simulink model "Boat_sim_HeadingHold"  (Simulink 7.5)
settings: Solver=FixedStepDiscrete  StartTime=0.0  StopTime=1000  FixedStep=.01  RelTol=1e-3
InitFcn:
  | boat_constants
values from neighbouring files (symbols this model uses):
  C_d_sea_surge = 340    [boat_constants.m]
  d_prop = .4572    (= 0.4572)    [boat_constants.m]
  figure8_waypoints = int32([ ... (first row only)    [boat_constants.m]
  K_t = 0.5    [boat_constants.m]
  mass = 550    [boat_constants.m]
  OC2max = 49999    [boat_constants.m]    (also in simulation_constants.m)
  phi_0 = 0    [boat_constants.m]    (also in simulation_constants.m)
  rho_w = 1.03e3    (= 1030)    [boat_constants.m]
  sampling_waypoints = int32([ ... (first row only)    [boat_constants.m]
  T_step = 0.01    [boat_constants.m]    (also in common.m)
  test_waypoints = int32([ ... (first row only)    [boat_constants.m]
  wheelbase = 3.27    [boat_constants.m]
undefined symbols (not defined in the file or in its folder): clock, DiscIntNeverNeededParam, Earth, WGS84
libraries: simulink x24, uSimLib x6, instrumentlib x2, aerolibconvert2 x2, aerolibtransform2 x1, aerolibanimutils x1, simulink_need_slupdate x1
(part 1 of 2)
settings Model: Creator=Administrator  LastModifiedBy=Bryant  ExtModeAutoUpdateStatusClock=off  BufferReuse=off
settings DataIOCC: MaxDataPoints=1  SaveOutput=off  SignalLogging=off  DSMLogging=off
settings OptimizationCC: BlockReduction=off  InlineParams=on  UseIntDivNetSlope=on  InlineInvariantSignals=on  BufferReuse=off  InitFltsAndDblsToZero=on  EfficientFloat2IntCast=on  SimCompilerOptimization=On
settings DebuggingCC: ReadBeforeWriteMsg=DisableAll  SaveWithParameterizedLinksMsg=none  FcnCallInpInsideContextMsg=Enable All  UniqueDataStoreMsg=error  AssertControl=DisableAll  StrictBusMsg=Warning
settings HardwareCC: ProdBitPerInt=16  ProdIntDivRoundTo=Zero  ProdEndianess=LittleEndian  ProdWordSize=16  ProdHWDeviceType=Microchip->dsPIC
settings GRTTargetCC: TargetFcnLib=ansi_tfl_tmw.mat

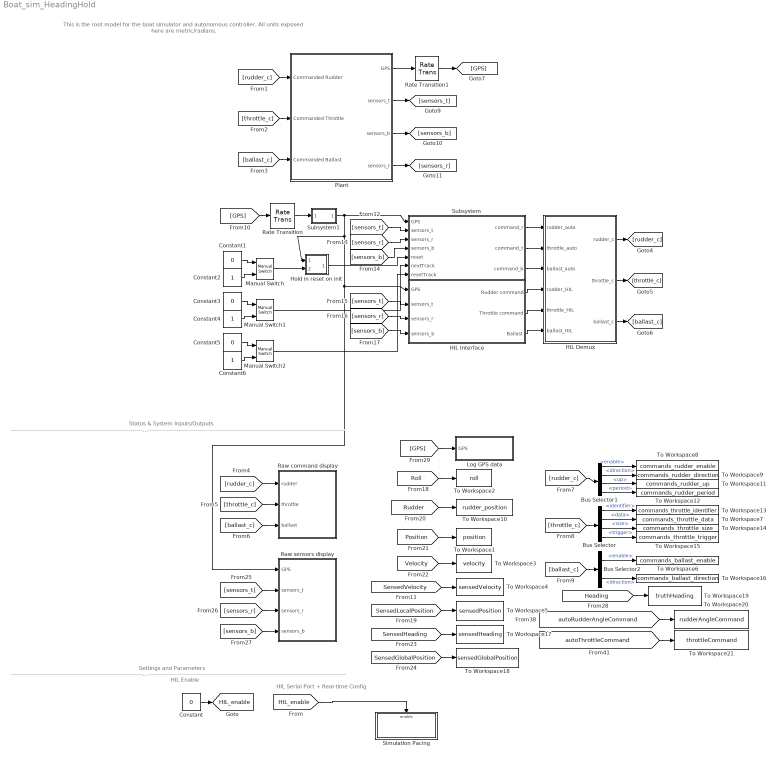
== system Boat_sim_HeadingHold ==
  note: This is the root model for the boat simulator and autonomous controller. All
      | units exposed here are metric/radians.
  note: HIL Enable
  note: Settings and Parameters
      | ---------------------------------------------------------------------------------------------------------------------------------------------------------------------------------------------------------------------------------------------------------
  note: HIL Serial Port + Real-time Config
  note: Status & System Inputs/Outputs
      | ---------------------------------------------------------------------------------------------------------------------------------------------------------------------------------------------------------------------------------------------------------
  Bus Selector : BusSelector  OutputSignals=identifier,data,size,trigger
  Bus Selector1 : BusSelector  OutputSignals=enable,direction,up,period
  Bus Selector2 : BusSelector  OutputSignals=enable,direction
  Constant : Constant  Value=0  OutDataTypeMode=boolean  OutDataType=fixdt(1, 16)  OutScaling=2^0  OutDataTypeStr=boolean
  Constant1 : Constant  Value=0  OutDataTypeMode=boolean  OutDataType=fixdt(1, 16)  OutScaling=2^0  OutDataTypeStr=boolean  SampleTime=Inf
  Constant2 : Constant  OutDataTypeMode=boolean  OutDataType=fixdt(1, 16)  OutScaling=2^0  OutDataTypeStr=boolean  SampleTime=Inf
  Constant3 : Constant  Value=0  OutDataTypeMode=boolean  OutDataType=fixdt(1, 16)  OutScaling=2^0  OutDataTypeStr=boolean  SampleTime=Inf
  Constant4 : Constant  OutDataTypeMode=boolean  OutDataType=fixdt(1, 16)  OutScaling=2^0  OutDataTypeStr=boolean  SampleTime=Inf
  Constant5 : Constant  Value=0  OutDataTypeMode=boolean  OutDataType=fixdt(1, 16)  OutScaling=2^0  OutDataTypeStr=boolean  SampleTime=Inf
  Constant6 : Constant  OutDataTypeMode=boolean  OutDataType=fixdt(1, 16)  OutScaling=2^0  OutDataTypeStr=boolean  SampleTime=Inf
  HIL Demux : Subsystem
  HIL Interface : Subsystem
  Hold in reset on init : Subsystem
  Log GPS data : Subsystem
  Manual Switch : simulink/Signal Routing/Manual Switch  SystemSampleTime=-1  sw=1  action=0  varsize=off
  Manual Switch1 : simulink/Signal Routing/Manual Switch  SystemSampleTime=-1  sw=1  action=0  varsize=off
  Manual Switch2 : simulink/Signal Routing/Manual Switch  SystemSampleTime=-1  sw=1  action=0  varsize=off
  Plant : Subsystem
  Rate Transition : RateTransition  Deterministic=off
  Rate Transition1 : RateTransition  Deterministic=off  OutPortSampleTime=1
  Raw command display : Subsystem
  Raw sensors display : Subsystem
  Simulation Pacing : Subsystem  TreatAsAtomicUnit=on
  Subsystem : Subsystem
  Subsystem1 : Subsystem
  To Workspace1 : ToWorkspace  VariableName=position  SampleTime=-1  SaveFormat=Array
  To Workspace10 : ToWorkspace  VariableName=rudder_position  SampleTime=-1  SaveFormat=Array
  To Workspace11 : ToWorkspace  VariableName=commands_rudder_up  SampleTime=-1  SaveFormat=Array
  To Workspace12 : ToWorkspace  VariableName=commands_rudder_period  SampleTime=-1  SaveFormat=Array
  To Workspace13 : ToWorkspace  VariableName=commands_throttle_identifier  SampleTime=-1  SaveFormat=Array
  To Workspace14 : ToWorkspace  VariableName=commands_throttle_size  SampleTime=-1  SaveFormat=Array
  To Workspace15 : ToWorkspace  VariableName=commands_throttle_trigger  SampleTime=-1  SaveFormat=Array
  To Workspace16 : ToWorkspace  VariableName=commands_ballast_direction  SampleTime=-1  SaveFormat=Array
  To Workspace17 : ToWorkspace  VariableName=sensedHeading  SampleTime=-1  SaveFormat=Array
  To Workspace18 : ToWorkspace  VariableName=sensedGlobalPosition  SampleTime=-1  SaveFormat=Array
  To Workspace19 : ToWorkspace  VariableName=truthHeading  SampleTime=-1  SaveFormat=Array
  To Workspace2 : ToWorkspace  VariableName=roll  SampleTime=-1  SaveFormat=Array
  To Workspace20 : ToWorkspace  VariableName=rudderAngleCommand  SampleTime=-1  SaveFormat=Array
  To Workspace21 : ToWorkspace  VariableName=throttleCommand  SampleTime=-1  SaveFormat=Array
  To Workspace3 : ToWorkspace  VariableName=velocity  SampleTime=-1  SaveFormat=Array
  To Workspace4 : ToWorkspace  VariableName=sensedVelocity  SampleTime=-1  SaveFormat=Array
  To Workspace5 : ToWorkspace  VariableName=sensedPosition  SampleTime=-1  SaveFormat=Array
  To Workspace6 : ToWorkspace  VariableName=commands_ballast_enable  SampleTime=-1  SaveFormat=Array
  To Workspace7 : ToWorkspace  VariableName=commands_throttle_data  SampleTime=-1  SaveFormat=Array
  To Workspace8 : ToWorkspace  VariableName=commands_rudder_enable  SampleTime=-1  SaveFormat=Array
  To Workspace9 : ToWorkspace  VariableName=commands_rudder_direction  SampleTime=-1  SaveFormat=Array
  tag scope: HIL_enable=global
  wires:
  Plant/4(sensors_r) -> [sensors_r]
  Constant/1 -> [HIL_enable]
  Subsystem/1(command_r) -> HIL Demux/1(rudder_auto)
  Subsystem/2(command_t) -> HIL Demux/2(throttle_auto)
  Subsystem/3(command_b) -> HIL Demux/3(ballast_auto)
  [rudder_c] -> Plant/1(Commanded Rudder)
  [throttle_c] -> Plant/2(Commanded Throttle)
  [ballast_c] -> Plant/3(Commanded Ballast)
  Plant/1(GPS) -> Rate Transition1/1
  Plant/3(sensors_b) -> [sensors_b]
  Plant/2(sensors_t) -> [sensors_t]
  [sensors_b] -> Subsystem/4(sensors_b)
  [sensors_r] -> Subsystem/3(sensors_r)
  [sensors_t] -> Subsystem/2(sensors_t)
  Constant1/1 -> Manual Switch/1
  Constant2/1 -> Manual Switch/2
  [rudder_c] -> Raw command display/1(rudder)
  [throttle_c] -> Raw command display/2(throttle)
  [ballast_c] -> Raw command display/3(ballast)
  [sensors_t] -> Raw sensors display/2(sensors_t)
  [sensors_r] -> Raw sensors display/3(sensors_r)
  [sensors_b] -> Raw sensors display/4(sensors_b)
  HIL Interface/1(Rudder command) -> HIL Demux/4(rudder_HIL)
  HIL Interface/2(Throttle command) -> HIL Demux/5(throttle_HIL)
  HIL Interface/3(Ballast) -> HIL Demux/6(ballast_HIL)
  HIL Demux/1(rudder_c) -> [rudder_c]
  HIL Demux/3(ballast_c) -> [ballast_c]
  HIL Demux/2(throttle_c) -> [throttle_c]
  [sensors_b] -> HIL Interface/4(sensors_b)
  [sensors_r] -> HIL Interface/3(sensors_r)
  [sensors_t] -> HIL Interface/2(sensors_t)
  [HIL_enable] -> Simulation Pacing/Enable
  [ballast_c] -> Bus Selector2/1
  [Roll] -> To Workspace2/1
  [Rudder] -> To Workspace10/1
  [Position] -> To Workspace1/1
  [throttle_c] -> Bus Selector/1
  Bus Selector/2 -> To Workspace7/1  "<data>"
  [rudder_c] -> Bus Selector1/1
  Bus Selector1/1 -> To Workspace8/1  "<enable>"
  [Velocity] -> To Workspace3/1
  Rate Transition/1 -> Subsystem1/1(GPS)
  Hold in reset on init/1(Out1) -> Subsystem/5(reset)
  Manual Switch/1 -> Hold in reset on init/2(reset)
  [GPS] -> Rate Transition/1
  Subsystem1/1(GPS+newData) -> Subsystem/1(GPS), Hold in reset on init/1(GPS), HIL Interface/1(GPS), Raw sensors display/1(GPS)
  Constant3/1 -> Manual Switch1/1
  Constant4/1 -> Manual Switch1/2
  Constant5/1 -> Manual Switch2/1
  Constant6/1 -> Manual Switch2/2
  Manual Switch2/1 -> Subsystem/7(resetTrack)
  Manual Switch1/1 -> Subsystem/6(nextTrack)
  [SensedVelocity] -> To Workspace4/1
  [SensedLocalPosition] -> To Workspace5/1
  Bus Selector1/2 -> To Workspace9/1  "<direction>"
  Bus Selector1/3 -> To Workspace11/1  "<up>"
  Bus Selector1/4 -> To Workspace12/1  "<period>"
  Bus Selector/1 -> To Workspace13/1  "<identifier>"
  Bus Selector/3 -> To Workspace14/1  "<size>"
  Bus Selector/4 -> To Workspace15/1  "<trigger>"
  Bus Selector2/1 -> To Workspace6/1  "<enable>"
  Bus Selector2/2 -> To Workspace16/1  "<direction>"
  [SensedHeading] -> To Workspace17/1
  [SensedGlobalPosition] -> To Workspace18/1
  [Heading] -> To Workspace19/1
  [autoRudderAngleCommand] -> To Workspace20/1
  [autoThrottleCommand] -> To Workspace21/1
  [GPS] -> Log GPS data/1(GPS)
  Rate Transition1/1 -> [GPS]

== system Boat_sim_HeadingHold/HIL Demux ==
  rudder_auto : Inport  OutDataType=fixdt(1, 16)  OutScaling=2^0
  throttle_auto : Inport  Port=2  OutDataType=fixdt(1, 16)  OutScaling=2^0
  ballast_auto : Inport  Port=3  OutDataType=fixdt(1, 16)  OutScaling=2^0
  rudder_HIL : Inport  Port=4  OutDataType=fixdt(1, 16)  OutScaling=2^0
  throttle_HIL : Inport  Port=5  OutDataType=fixdt(1, 16)  OutScaling=2^0
  ballast_HIL : Inport  Port=6  OutDataType=fixdt(1, 16)  OutScaling=2^0
  Switch : Switch  Criteria=u2 ~= 0  OutDataType=fixdt(1, 16)  OutScaling=2^0
  Switch1 : Switch  Criteria=u2 ~= 0  OutDataType=fixdt(1, 16)  OutScaling=2^0
  Switch2 : Switch  Criteria=u2 ~= 0  OutDataType=fixdt(1, 16)  OutScaling=2^0
  rudder_c : Outport  OutDataType=fixdt(1, 16)  OutScaling=2^0
  throttle_c : Outport  Port=2  OutDataType=fixdt(1, 16)  OutScaling=2^0
  ballast_c : Outport  Port=3  OutDataType=fixdt(1, 16)  OutScaling=2^0
  wires:
  rudder_HIL/1 -> Switch/1
  [HIL_enable] -> Switch/2, Switch1/2, Switch2/2
  throttle_HIL/1 -> Switch1/1
  ballast_HIL/1 -> Switch2/1
  throttle_auto/1 -> Switch1/3
  rudder_auto/1 -> Switch/3
  ballast_auto/1 -> Switch2/3
  Switch/1 -> rudder_c/1
  Switch1/1 -> throttle_c/1
  Switch2/1 -> ballast_c/1

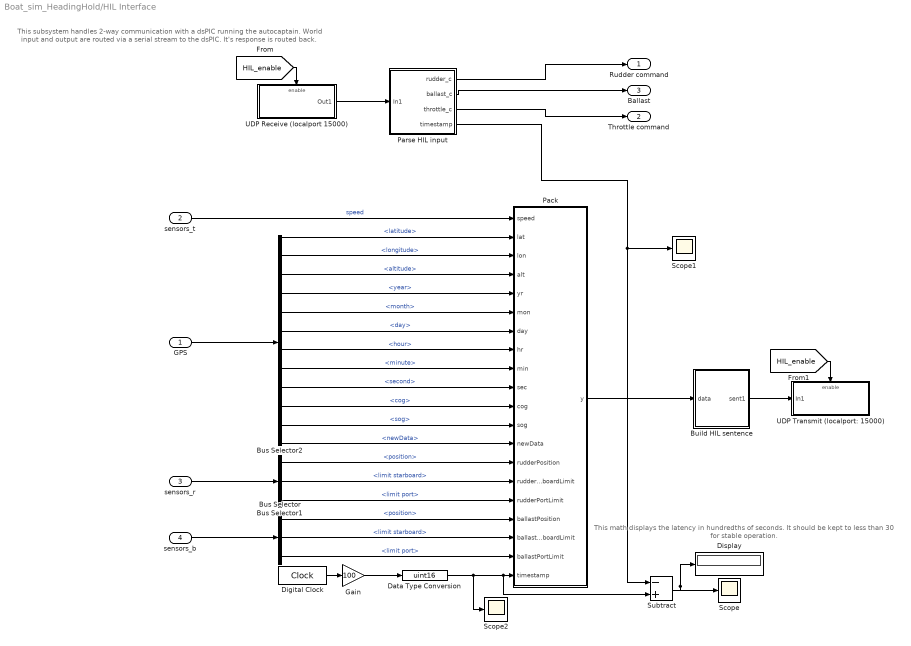
== system Boat_sim_HeadingHold/HIL Interface ==
  note: This subsystem handles 2-way communication with a dsPIC running
      | the autocaptain. World input and output are routed via a serial stream
      | to the dsPIC. It's response is routed back.
  note: This math displays the latency in hundredths of seconds.
      | It should be kept to less than 30 for stable operation.
  GPS : Inport  OutDataType=fixdt(1, 16)  OutScaling=2^0
  sensors_t : Inport  Port=2  OutDataType=fixdt(1, 16)  OutScaling=2^0
  sensors_r : Inport  Port=3  OutDataType=fixdt(1, 16)  OutScaling=2^0
  sensors_b : Inport  Port=4  OutDataType=fixdt(1, 16)  OutScaling=2^0
  Build HIL sentence : Subsystem
  Bus Selector : BusSelector  OutputSignals=position,limit starboard,limit port
  Bus Selector1 : BusSelector  OutputSignals=position,limit starboard,limit port
  Bus Selector2 : BusSelector  OutputSignals=latitude,longitude,altitude,year,month,day,hour,minute,second,cog,sog,newData
  Data Type Conversion : DataTypeConversion  OutDataTypeMode=uint16  OutDataType=fixdt(1, 16)  OutScaling=2^0  OutDataTypeStr=uint16
  Digital Clock : DigitalClock  SampleTime=.01
  Display : Display
  Gain : Gain  Gain=100  ParameterDataType=fixdt(1, 16)  ParameterScaling=2^0  OutDataType=fixdt(1, 16)  OutScaling=2^0
  Pack : Stateflow chart  TreatAsAtomicUnit=on
  Parse HIL input : Subsystem
  Scope : Scope
      settings: YMin=40  YMax=92.5  SaveName=latency  DataFormat=Array
  Scope1 : Scope
      settings: YMin=1470.6  YMax=1625.4  SaveName=latency_in  DataFormat=Array
  Scope2 : Scope
      settings: TimeRange=14  YMin=0  YMax=1400  SaveName=latency_out  DataFormat=Array
  Subtract : Sum  Inputs=-+  OutDataTypeMode=int16  OutDataType=fixdt(1, 16)  OutScaling=2^-10  OutDataTypeStr=int16
  UDP Receive (localport 15000) : Subsystem  TreatAsAtomicUnit=on
  UDP Transmit (localport: 15000) : Subsystem  TreatAsAtomicUnit=on
  Rudder command : Outport  OutDataType=fixdt(1, 16)  OutScaling=2^0
  Throttle command : Outport  Port=2  OutDataType=fixdt(1, 16)  OutScaling=2^0
  Ballast : Outport  Port=3  OutDataType=fixdt(1, 16)  OutScaling=2^0
  wires:
  UDP Receive (localport 15000)/1(Out1) -> Parse HIL input/1(In1)
  Parse HIL input/2(ballast_c) -> Ballast/1
  Parse HIL input/1(rudder_c) -> Rudder command/1
  sensors_b/1 -> Bus Selector/1
  sensors_r/1 -> Bus Selector1/1
  GPS/1 -> Bus Selector2/1
  Parse HIL input/3(throttle_c) -> Throttle command/1
  Pack/1(y) -> Build HIL sentence/1(data)
  sensors_t/1 -> Pack/1(speed)  "speed"
  Bus Selector2/1 -> Pack/2(lat)  "<latitude>"
  Bus Selector2/2 -> Pack/3(lon)  "<longitude>"
  Bus Selector2/3 -> Pack/4(alt)  "<altitude>"
  Bus Selector2/4 -> Pack/5(yr)  "<year>"
  Bus Selector2/5 -> Pack/6(mon)  "<month>"
  Bus Selector2/6 -> Pack/7(day)  "<day>"
  Bus Selector2/7 -> Pack/8(hr)  "<hour>"
  Bus Selector2/8 -> Pack/9(min)  "<minute>"
  Bus Selector2/9 -> Pack/10(sec)  "<second>"
  Bus Selector2/10 -> Pack/11(cog)  "<cog>"
  Bus Selector2/11 -> Pack/12(sog)  "<sog>"
  [HIL_enable] -> UDP Receive (localport 15000)/Enable
  [HIL_enable] -> UDP Transmit (localport: 15000)/Enable
  Build HIL sentence/1(sent1) -> UDP Transmit (localport: 15000)/1(In1)
  Parse HIL input/4(timestamp) -> Subtract/1, Scope1/1
  Gain/1 -> Data Type Conversion/1
  Digital Clock/1 -> Gain/1
  Data Type Conversion/1 -> Subtract/2, Pack/20(timestamp), Scope2/1
  Subtract/1 -> Scope/1, Display/1
  Bus Selector2/12 -> Pack/13(newData)  "<newData>"
  Bus Selector1/1 -> Pack/14(rudderPosition)  "<position>"
  Bus Selector1/2 -> Pack/15(rudderStarboardLimit)  "<limit starboard>"
  Bus Selector1/3 -> Pack/16(rudderPortLimit)  "<limit port>"
  Bus Selector/1 -> Pack/17(ballastPosition)  "<position>"
  Bus Selector/2 -> Pack/18(ballastStarboardLimit)  "<limit starboard>"
  Bus Selector/3 -> Pack/19(ballastPortLimit)  "<limit port>"

== system Boat_sim_HeadingHold/Hold in reset on init ==
  GPS : Inport
  reset : Inport  Port=2
  Bus Selector : BusSelector  OutputSignals=newData
  Compare To Zero : simulink/Logic and Bit Operations/Compare To Zero  SystemSampleTime=-1  relop===  LogicOutDataTypeMode=uint8
  Discrete-Time Integrator : DiscreteIntegrator  SampleTime=-1  OutDataType=fixdt(1, 16)  OutScaling=2^0  LimitOutput=on  UpperSaturationLimit=1  LowerSaturationLimit=0  ICPrevOutput=DiscIntNeverNeededParam  ICPrevScaledInput=DiscIntNeverNeededParam
  Logical Operator : Logic  Operator=OR  AllPortsSameDT=off  OutDataTypeMode=boolean  LogicDataType=fixdt(0, 8)  OutDataTypeStr=boolean
  Out1 : Outport
  wires:
  Bus Selector/1 -> Discrete-Time Integrator/1  "<newData>"
  Discrete-Time Integrator/1 -> Compare To Zero/1
  Compare To Zero/1 -> Logical Operator/1
  GPS/1 -> Bus Selector/1
  Logical Operator/1 -> Out1/1
  reset/1 -> Logical Operator/2

== system Boat_sim_HeadingHold/Log GPS data ==
  GPS : Inport
  Bus Selector3 : BusSelector  OutputSignals=latitude,longitude,altitude,year,month,day,hour,minute,second,cog,sog
  Mux : Mux  Inputs=3
  To Workspace22 : ToWorkspace  VariableName=gpsMonth  SampleTime=-1  SaveFormat=Array
  To Workspace23 : ToWorkspace  VariableName=gpsDay  SampleTime=-1  SaveFormat=Array
  To Workspace24 : ToWorkspace  VariableName=gpsHour  SampleTime=-1  SaveFormat=Array
  To Workspace25 : ToWorkspace  VariableName=gpsYear  SampleTime=-1  SaveFormat=Array
  To Workspace26 : ToWorkspace  VariableName=gpsMinute  SampleTime=-1  SaveFormat=Array
  To Workspace27 : ToWorkspace  VariableName=gpsSecond  SampleTime=-1  SaveFormat=Array
  To Workspace28 : ToWorkspace  VariableName=globalPosition  SampleTime=-1  SaveFormat=Array
  To Workspace29 : ToWorkspace  VariableName=courseOverGround  SampleTime=-1  SaveFormat=Array
  To Workspace30 : ToWorkspace  VariableName=speedOverGround  SampleTime=-1  SaveFormat=Array
  wires:
  Mux/1 -> To Workspace28/1
  Bus Selector3/1 -> Mux/1  "<latitude>"
  Bus Selector3/2 -> Mux/2  "<longitude>"
  Bus Selector3/3 -> Mux/3  "<altitude>"
  Bus Selector3/4 -> To Workspace25/1  "<year>"
  Bus Selector3/5 -> To Workspace22/1  "<month>"
  Bus Selector3/6 -> To Workspace23/1  "<day>"
  Bus Selector3/7 -> To Workspace24/1  "<hour>"
  Bus Selector3/8 -> To Workspace26/1  "<minute>"
  Bus Selector3/9 -> To Workspace27/1  "<second>"
  Bus Selector3/10 -> To Workspace29/1  "<cog>"
  Bus Selector3/11 -> To Workspace30/1  "<sog>"
  GPS/1 -> Bus Selector3/1

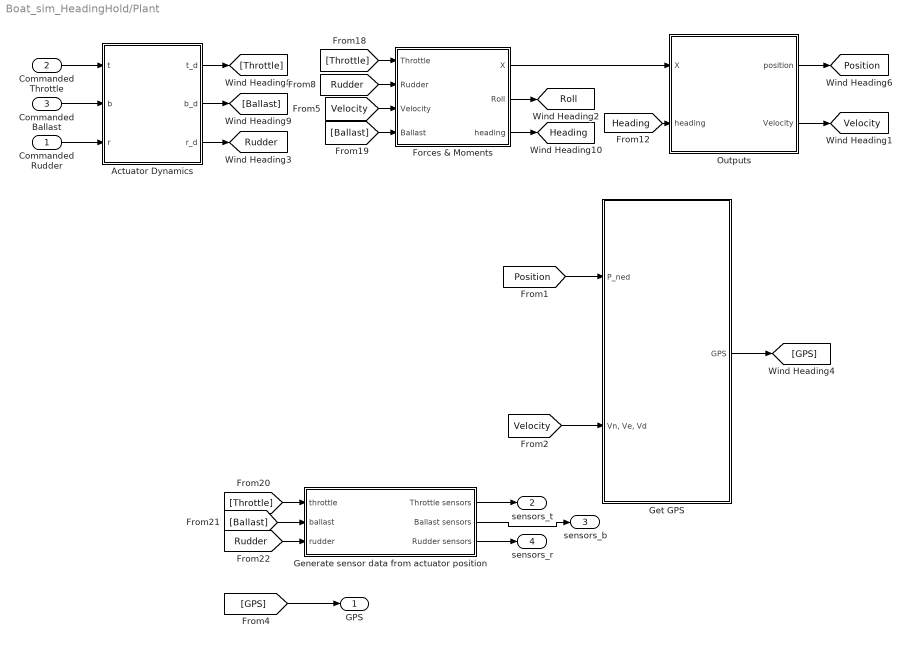
== system Boat_sim_HeadingHold/Plant ==
  Commanded Rudder : Inport  OutDataType=sfix(16)  OutScaling=2^0
  Commanded Throttle : Inport  Port=2  OutDataType=sfix(16)  OutScaling=2^0
  Commanded Ballast : Inport  Port=3  OutDataType=sfix(16)  OutScaling=2^0
  Actuator Dynamics : Subsystem
  Forces & Moments : Subsystem
  Generate sensor data from actuator position : Subsystem
  Get GPS : Subsystem
  Outputs : Subsystem
  GPS : Outport  OutDataType=sfix(16)  OutScaling=2^0
  sensors_t : Outport  Port=2  OutDataType=sfix(16)  OutScaling=2^0
  sensors_b : Outport  Port=3  OutDataType=sfix(16)  OutScaling=2^0
  sensors_r : Outport  Port=4  OutDataType=sfix(16)  OutScaling=2^0
  tag scope: Heading=global, Position=global, Roll=global, Rudder=global, Velocity=global
  wires:
  Forces & Moments/1(X) -> Outputs/1(X)
  Commanded Throttle/1 -> Actuator Dynamics/1(t)
  Commanded Rudder/1 -> Actuator Dynamics/3(r)
  Forces & Moments/2(Roll) -> [Roll]
  Commanded Ballast/1 -> Actuator Dynamics/2(b)
  [Velocity] -> Forces & Moments/3(Velocity)
  Actuator Dynamics/3(r_d) -> [Rudder]
  [Rudder] -> Forces & Moments/2(Rudder)
  [Heading] -> Outputs/2(heading)
  Actuator Dynamics/1(t_d) -> [Throttle]
  [Throttle] -> Forces & Moments/1(Throttle)
  [Ballast] -> Forces & Moments/4(Ballast)
  Actuator Dynamics/2(b_d) -> [Ballast]
  Forces & Moments/3(heading) -> [Heading]
  Outputs/2(Velocity) -> [Velocity]
  Outputs/1(position) -> [Position]
  [Position] -> Get GPS/1(P_ned)
  [Velocity] -> Get GPS/2("Vn, Ve, Vd")
  Get GPS/1(GPS) -> [GPS]
  [GPS] -> GPS/1
  [Rudder] -> Generate sensor data from actuator position/3(rudder)
  [Ballast] -> Generate sensor data from actuator position/2(ballast)
  [Throttle] -> Generate sensor data from actuator position/1(throttle)
  Generate sensor data from actuator position/1(Throttle sensors) -> sensors_t/1
  Generate sensor data from actuator position/2(Ballast sensors) -> sensors_b/1
  Generate sensor data from actuator position/3(Rudder sensors) -> sensors_r/1

== system Boat_sim_HeadingHold/Raw command display ==
  rudder : Inport
  throttle : Inport  Port=2
  ballast : Inport  Port=3
  Bus Selector3 : BusSelector  OutputSignals=enable,direction,up,period
  Bus Selector4 : BusSelector  OutputSignals=identifier,data,size,trigger
  Bus Selector5 : BusSelector  OutputSignals=enable,direction
  Display{,1..9} (10 alike) : Display
      Display4 settings: Format=hex (Stored Integer)
      Display5 settings: Format=hex (Stored Integer)
  wires:
  Bus Selector3/4 -> Display3/1  "<period>"
  Bus Selector3/1 -> Display/1  "<enable>"
  Bus Selector3/2 -> Display1/1  "<direction>"
  Bus Selector3/3 -> Display2/1  "<up>"
  Bus Selector4/4 -> Display7/1  "<trigger>"
  Bus Selector4/1 -> Display4/1  "<identifier>"
  Bus Selector4/2 -> Display5/1  "<data>"
  Bus Selector4/3 -> Display6/1  "<size>"
  Bus Selector5/2 -> Display8/1  "<direction>"
  Bus Selector5/1 -> Display9/1  "<enable>"
  rudder/1 -> Bus Selector3/1
  throttle/1 -> Bus Selector4/1
  ballast/1 -> Bus Selector5/1

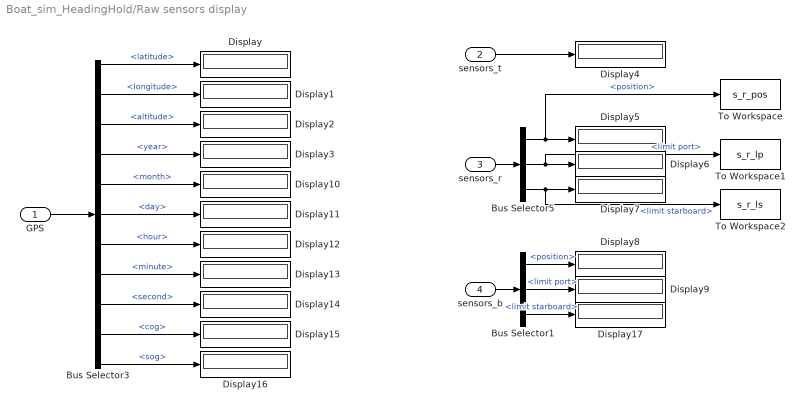
== system Boat_sim_HeadingHold/Raw sensors display ==
  GPS : Inport
  sensors_t : Inport  Port=2
  sensors_r : Inport  Port=3
  sensors_b : Inport  Port=4
  Bus Selector1 : BusSelector  OutputSignals=position,limit port,limit starboard
  Bus Selector3 : BusSelector  OutputSignals=latitude,longitude,altitude,year,month,day,hour,minute,second,cog,sog
  Bus Selector5 : BusSelector  OutputSignals=position,limit port,limit starboard
  Display{,1..17} (18 alike) : Display
  To Workspace : ToWorkspace  VariableName=s_r_pos  SampleTime=-1  SaveFormat=Array
  To Workspace1 : ToWorkspace  VariableName=s_r_lp  SampleTime=-1  SaveFormat=Array
  To Workspace2 : ToWorkspace  VariableName=s_r_ls  SampleTime=-1  SaveFormat=Array
  wires:
  Bus Selector3/4 -> Display3/1  "<year>"
  Bus Selector3/1 -> Display/1  "<latitude>"
  Bus Selector3/2 -> Display1/1  "<longitude>"
  Bus Selector3/3 -> Display2/1  "<altitude>"
  GPS/1 -> Bus Selector3/1
  sensors_t/1 -> Display4/1
  sensors_r/1 -> Bus Selector5/1
  Bus Selector3/5 -> Display10/1  "<month>"
  Bus Selector3/6 -> Display11/1  "<day>"
  Bus Selector3/7 -> Display12/1  "<hour>"
  Bus Selector3/8 -> Display13/1  "<minute>"
  Bus Selector3/9 -> Display14/1  "<second>"
  Bus Selector3/10 -> Display15/1  "<cog>"
  Bus Selector3/11 -> Display16/1  "<sog>"
  sensors_b/1 -> Bus Selector1/1
  Bus Selector5/1 -> Display5/1, To Workspace/1  "<position>"
  Bus Selector5/2 -> Display6/1, To Workspace1/1  "<limit port>"
  Bus Selector5/3 -> Display7/1, To Workspace2/1  "<limit starboard>"
  Bus Selector1/1 -> Display8/1  "<position>"
  Bus Selector1/2 -> Display9/1  "<limit port>"
  Bus Selector1/3 -> Display17/1  "<limit starboard>"

== system Boat_sim_HeadingHold/Simulation Pacing ==
  note: This block attempts to lock the simulation down to real-time. This does, however, require that the sim run faster than real time originally,
      | then the Set Pace block sleeps the MATLAB  process to fill up the time til it paces realtime. The number in the display block shouldn't be
      | far from 0 and will probably bounce around both above and below. If it stays substantially below zero (<-.01), then there's a problem as
      | the sim isn't keeping time.
  Enable : EnablePort
  Display1 : Display
      settings: Decimation=20
  Scope : Scope
      settings: SaveName=paceError  DataFormat=Array
  Simulation Pace : aerolibanimutils/Simulation Pace  SimulationPace=1  SleepMode=MATLAB Thread  OutputPaceError=on  SampleTime=T_step
      settings: AttributesFormatString=%<SimulationPace> sec/sec
  wires:
  Simulation Pace/1 -> Display1/1, Scope/1

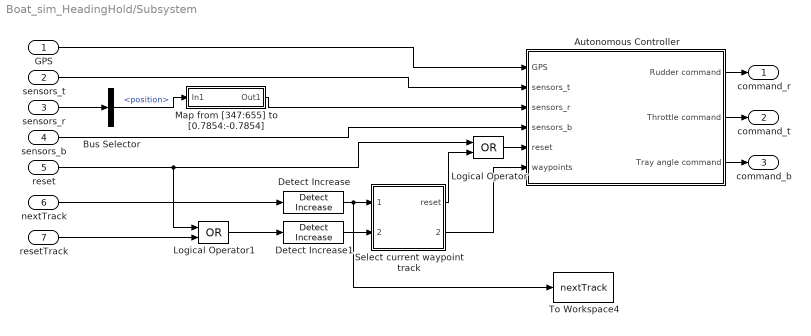
== system Boat_sim_HeadingHold/Subsystem ==
  GPS : Inport
  sensors_t : Inport  Port=2
  sensors_r : Inport  Port=3
  sensors_b : Inport  Port=4
  reset : Inport  Port=5
  nextTrack : Inport  Port=6
  resetTrack : Inport  Port=7
  Autonomous Controller : Subsystem
  Bus Selector : BusSelector  OutputSignals=position
  Detect Increase : simulink/Logic and Bit Operations/Detect Increase  SystemSampleTime=-1  vinit=0.0
  Detect Increase1 : simulink/Logic and Bit Operations/Detect Increase  SystemSampleTime=-1  vinit=0.0
  Logical Operator : Logic  Operator=OR  AllPortsSameDT=off  OutDataTypeMode=boolean  LogicDataType=fixdt(0, 8)  OutDataTypeStr=boolean
  Logical Operator1 : Logic  Operator=OR  AllPortsSameDT=off  OutDataTypeMode=boolean  LogicDataType=fixdt(0, 8)  OutDataTypeStr=boolean
  Map from [347:655] to [0.7854:-0.7854] : Subsystem
  Select current waypoint track : Stateflow chart  TreatAsAtomicUnit=on
  To Workspace4 : ToWorkspace  VariableName=nextTrack  SampleTime=-1  SaveFormat=Array
  command_r : Outport
  command_t : Outport  Port=2
  command_b : Outport  Port=3
  wires:
  GPS/1 -> Autonomous Controller/1(GPS)
  Autonomous Controller/1(Rudder command) -> command_r/1
  sensors_t/1 -> Autonomous Controller/2(sensors_t)
  sensors_r/1 -> Bus Selector/1
  Autonomous Controller/2(Throttle command) -> command_t/1
  sensors_b/1 -> Autonomous Controller/4(sensors_b)
  Autonomous Controller/3(Tray angle command) -> command_b/1
  nextTrack/1 -> Detect Increase/1
  Select current waypoint track/2(waypoints) -> Autonomous Controller/6(waypoints)
  Logical Operator/1 -> Autonomous Controller/5(reset)
  Select current waypoint track/1(reset) -> Logical Operator/2
  reset/1 -> Logical Operator/1, Logical Operator1/1
  Detect Increase/1 -> Select current waypoint track/1(nextTrack), To Workspace4/1
  Detect Increase1/1 -> Select current waypoint track/2(resetTrackNumber)
  Logical Operator1/1 -> Detect Increase1/1
  resetTrack/1 -> Logical Operator1/2
  Map from [347:655] to [0.7854:-0.7854]/1(Out1) -> Autonomous Controller/3(sensors_r)
  Bus Selector/1 -> Map from [347:655] to [0.7854:-0.7854]/1(In1)  "<position>"

== system Boat_sim_HeadingHold/Subsystem1 ==
  GPS : Inport
  Bus Creator : BusCreator  Inputs=12
  Bus Selector : BusSelector  OutputSignals=latitude,longitude,altitude,year,month,day,hour,minute,second,cog,sog
  Data Type Conversion : DataTypeConversion  OutDataTypeMode=boolean  OutDataType=fixdt(1, 16)  OutScaling=2^0  OutDataTypeStr=boolean
  Pulse Generator : DiscretePulseGenerator  Amplitude=1  Period=100  PulseWidth=1  PhaseDelay=100  SampleTime=T_step
  GPS+newData : Outport
  wires:
  Bus Selector/1 -> Bus Creator/1  "<latitude>"
  Bus Selector/2 -> Bus Creator/2  "<longitude>"
  Bus Selector/3 -> Bus Creator/3  "<altitude>"
  Bus Selector/4 -> Bus Creator/4  "<year>"
  Bus Selector/5 -> Bus Creator/5  "<month>"
  Bus Selector/6 -> Bus Creator/6  "<day>"
  Bus Selector/7 -> Bus Creator/7  "<hour>"
  Bus Selector/8 -> Bus Creator/8  "<minute>"
  Bus Selector/9 -> Bus Creator/9  "<second>"
  Bus Selector/10 -> Bus Creator/10  "<cog>"
  Bus Selector/11 -> Bus Creator/11  "<sog>"
  Pulse Generator/1 -> Data Type Conversion/1
  Data Type Conversion/1 -> Bus Creator/12  "newData"
  GPS/1 -> Bus Selector/1
  Bus Creator/1 -> GPS+newData/1

== system Boat_sim_HeadingHold/HIL Interface/Build HIL sentence ==
  data : Inport
  Bitwise Operator1 : simulink/Logic and Bit Operations/Bitwise Operator  logicop=XOR  UseBitMask=off  BitMask=bin2dec('11011001')  BitMaskRealWorld=Stored Integer
  Constant5 : Constant  Value=37  OutDataTypeMode=uint8  OutDataType=fixdt(1, 16)  OutScaling=2^0  OutDataTypeStr=uint8
  Constant6 : Constant  Value=38  OutDataTypeMode=uint8  OutDataType=fixdt(1, 16)  OutScaling=2^0  OutDataTypeStr=uint8
  Constant7 : Constant  Value=94  OutDataTypeMode=uint8  OutDataType=fixdt(1, 16)  OutScaling=2^0  OutDataTypeStr=uint8
  Constant8 : Constant  Value=38  OutDataTypeMode=uint8  OutDataType=fixdt(1, 16)  OutScaling=2^0  OutDataTypeStr=uint8
  Constant9 : Constant  OutDataTypeMode=uint8  OutDataType=fixdt(1, 16)  OutScaling=2^0  OutDataTypeStr=uint8
  Mux3 : Mux  Inputs=3
  Pack : Stateflow chart  TreatAsAtomicUnit=on
  Probe : Probe  ProbeSampleTime=off  ProbeComplexSignal=off  ProbeWidthDataType=uint8
  sent1 : Outport
  wires:
  data/1 -> Probe/1, Mux3/3
  Constant5/1 -> Pack/1(a)
  Constant6/1 -> Pack/2(b)
  Pack/1(y) -> sent1/1
  Mux3/1 -> Bitwise Operator1/1, Pack/3(c)
  Probe/1 -> Mux3/2
  Constant7/1 -> Pack/4(d)
  Constant8/1 -> Pack/5(e)
  Bitwise Operator1/1 -> Pack/6(f)
  Constant9/1 -> Mux3/1

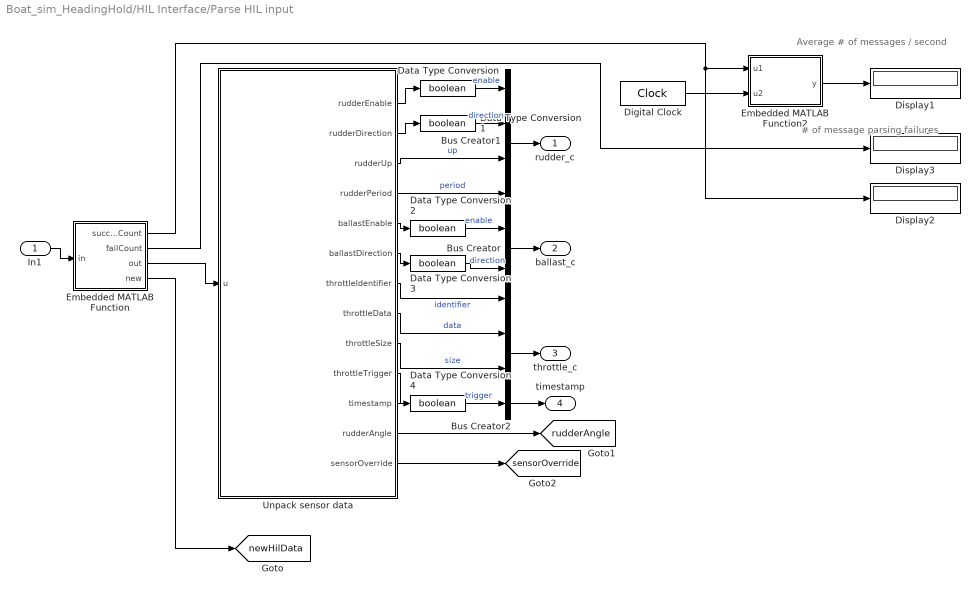
== system Boat_sim_HeadingHold/HIL Interface/Parse HIL input ==
  note: # of message parsing failures
  note: Average # of messages / second
  In1 : Inport
  Bus Creator : BusCreator  Inputs=2
  Bus Creator1 : BusCreator
  Bus Creator2 : BusCreator
  Data Type Conversion{,1..4} (5 alike) : DataTypeConversion  OutDataTypeMode=boolean  OutDataType=fixdt(1, 16)  OutScaling=2^0  OutDataTypeStr=boolean
  Digital Clock : DigitalClock  SampleTime=T_step
  Display1 : Display
  Display2 : Display
  Display3 : Display
  Embedded MATLAB Function : Stateflow chart  TreatAsAtomicUnit=on
  Embedded MATLAB Function2 : Stateflow chart  TreatAsAtomicUnit=on
  Unpack sensor data : Stateflow chart  TreatAsAtomicUnit=on
  rudder_c : Outport
  ballast_c : Outport  Port=2
  throttle_c : Outport  Port=3
  timestamp : Outport  Port=4
  tag scope: newHilData=global, rudderAngle=global, sensorOverride=global
  wires:
  Embedded MATLAB Function/3(out) -> Unpack sensor data/1(u)
  Bus Creator1/1 -> rudder_c/1
  In1/1 -> Embedded MATLAB Function/1(in)
  Bus Creator/1 -> ballast_c/1
  Bus Creator2/1 -> throttle_c/1
  Unpack sensor data/1(rudderEnable) -> Data Type Conversion/1
  Unpack sensor data/2(rudderDirection) -> Data Type Conversion1/1
  Unpack sensor data/3(rudderUp) -> Bus Creator1/3  "up"
  Unpack sensor data/4(rudderPeriod) -> Bus Creator1/4  "period"
  Unpack sensor data/5(ballastEnable) -> Data Type Conversion2/1
  Unpack sensor data/6(ballastDirection) -> Data Type Conversion3/1
  Unpack sensor data/7(throttleIdentifier) -> Bus Creator2/1  "identifier"
  Unpack sensor data/8(throttleData) -> Bus Creator2/2  "data"
  Unpack sensor data/9(throttleSize) -> Bus Creator2/3  "size"
  Unpack sensor data/10(throttleTrigger) -> Data Type Conversion4/1
  Unpack sensor data/11(timestamp) -> timestamp/1
  Embedded MATLAB Function/1(successCount) -> Embedded MATLAB Function2/1(u1), Display2/1
  Digital Clock/1 -> Embedded MATLAB Function2/2(u2)
  Embedded MATLAB Function2/1(y) -> Display1/1
  Data Type Conversion/1 -> Bus Creator1/1  "enable"
  Data Type Conversion1/1 -> Bus Creator1/2  "direction"
  Data Type Conversion2/1 -> Bus Creator/1  "enable"
  Data Type Conversion3/1 -> Bus Creator/2  "direction"
  Data Type Conversion4/1 -> Bus Creator2/4  "trigger"
  Embedded MATLAB Function/2(failCount) -> Display3/1
  Unpack sensor data/12(rudderAngle) -> [rudderAngle]
  Embedded MATLAB Function/4(new) -> [newHilData]
  Unpack sensor data/13(sensorOverride) -> [sensorOverride]

== system Boat_sim_HeadingHold/HIL Interface/UDP Receive (localport 15000) ==
  Enable : EnablePort
  Terminator : Terminator
  UDP Receive : instrumentlib/UDP Receive  DialogController=instrumentcreatedialog  DialogControllerArgs=DataTag0  Host=127.0.0.1  Port=15000  LocalPort=16000  DataSize=34  EnableBlockingMode=off  Timeout=10  SampleTime=0.01  DataType=uint8  ByteOrder=BigEndian
  Out1 : Outport  OutDataType=fixdt(1, 16)  OutScaling=2^0
  wires:
  UDP Receive/1 -> Out1/1
  UDP Receive/2 -> Terminator/1

== system Boat_sim_HeadingHold/HIL Interface/UDP Transmit (localport: 15000) ==
  note: This subsystem transmits the necessary data to the dsPIC.
  In1 : Inport  OutDataType=fixdt(1, 16)  OutScaling=2^0
  Enable : EnablePort
  UDP Send : instrumentlib/UDP Send  DialogController=instrumentcreatedialog  DialogControllerArgs=DataTag1  Host=127.0.0.1  Port=15000  LocalPort=16000  EnableBlockingMode=on  ByteOrder=BigEndian
  wires:
  In1/1 -> UDP Send/1

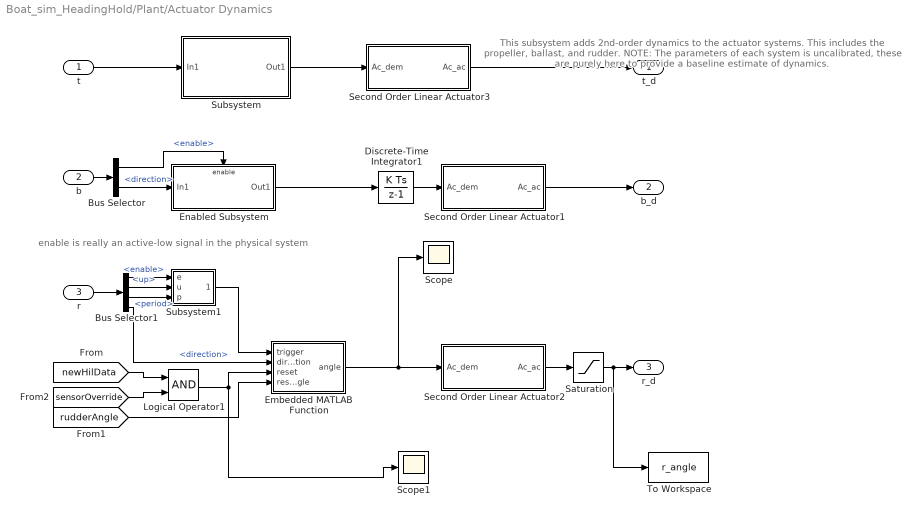
== system Boat_sim_HeadingHold/Plant/Actuator Dynamics ==
  note: This subsystem adds 2nd-order dynamics to the actuator systems.
      | This includes the propeller, ballast, and rudder.
      |
      | NOTE: The parameters of each system is uncalibrated, these are
      | purely here to provide a baseline estimate of dynamics.
  note: enable is really an active-low signal
      | in the physical system
  t : Inport  OutDataType=sfix(16)  OutScaling=2^0
  b : Inport  Port=2  OutDataType=sfix(16)  OutScaling=2^0
  r : Inport  Port=3  OutDataType=sfix(16)  OutScaling=2^0
  Bus Selector : BusSelector  OutputSignals=enable,direction
  Bus Selector1 : BusSelector  OutputSignals=enable,up,period,direction
  Discrete-Time Integrator1 : DiscreteIntegrator  SampleTime=-1  OutDataType=fixdt(1, 16)  OutScaling=2^0  UpperSaturationLimit=1  LowerSaturationLimit=-1  ICPrevOutput=DiscIntNeverNeededParam  ICPrevScaledInput=DiscIntNeverNeededParam
  Embedded MATLAB Function : Stateflow chart  TreatAsAtomicUnit=on
  Enabled Subsystem : Subsystem  TreatAsAtomicUnit=on
  Logical Operator1 : Logic  AllPortsSameDT=off  OutDataTypeMode=boolean  LogicDataType=fixdt(0, 8)  OutDataTypeStr=boolean
  Saturation : Saturate  UpperLimit=.7854  LowerLimit=-.7854  OutDataType=fixdt(1, 16)  OutScaling=2^0
  Scope : Scope
      settings: SaveName=rudderChange  DataFormat=Array
  Scope1 : Scope
      settings: SaveName=rudderChange1  DataFormat=Array
  Second Order Linear Actuator1 : Subsystem  AncestorBlock=aerolibactuator/Second Order Linear Actuator  mask(Second Order Linear Actuator){wn_fin=15, z_fin=0.8, fin_act_0=0}
      mask prompts: wn_fin "Natural frequency:"; z_fin "Damping ratio:"; fin_act_0 "Initial position:"
      mask help: Implement a second-order actuator model
      mask init:
      | aeroicon('aeroblk');
      mask Help: eval('asbhelp');
      mask Display:
      | port_label('input',1,'A_{demand}','texmode','on');
      | port_label('output',1,'A_{actual}','texmode','on');
  Second Order Linear Actuator2 : Subsystem  AncestorBlock=aerolibactuator/Second Order Linear Actuator  mask(Second Order Linear Actuator){wn_fin=15, z_fin=0.8, fin_act_0=0}
      mask prompts: wn_fin "Natural frequency:"; z_fin "Damping ratio:"; fin_act_0 "Initial position:"
      mask help: Implement a second-order actuator model
      mask init:
      | aeroicon('aeroblk');
      mask Help: eval('asbhelp');
      mask Display:
      | port_label('input',1,'A_{demand}','texmode','on');
      | port_label('output',1,'A_{actual}','texmode','on');
  Second Order Linear Actuator3 : Subsystem  AncestorBlock=aerolibactuator/Second Order Linear Actuator  mask(Second Order Linear Actuator){wn_fin=15, z_fin=0.8, fin_act_0=0}
      mask prompts: wn_fin "Natural frequency:"; z_fin "Damping ratio:"; fin_act_0 "Initial position:"
      mask help: Implement a second-order actuator model
      mask init:
      | aeroicon('aeroblk');
      mask Help: eval('asbhelp');
      mask Display:
      | port_label('input',1,'A_{demand}','texmode','on');
      | port_label('output',1,'A_{actual}','texmode','on');
  Subsystem : Subsystem
  Subsystem1 : Subsystem
  To Workspace : ToWorkspace  VariableName=r_angle  SampleTime=-1  SaveFormat=Array
  t_d : Outport  OutDataType=sfix(16)  OutScaling=2^0
  b_d : Outport  Port=2  OutDataType=sfix(16)  OutScaling=2^0
  r_d : Outport  Port=3  OutDataType=sfix(16)  OutScaling=2^0
  wires:
  r/1 -> Bus Selector1/1
  Second Order Linear Actuator1/1(Ac_ac) -> b_d/1
  Embedded MATLAB Function/1(angle) -> Second Order Linear Actuator2/1(Ac_dem), Scope/1
  Subsystem/1(Out1) -> Second Order Linear Actuator3/1(Ac_dem)
  b/1 -> Bus Selector/1
  Enabled Subsystem/1(Out1) -> Discrete-Time Integrator1/1
  Discrete-Time Integrator1/1 -> Second Order Linear Actuator1/1(Ac_dem)
  Bus Selector/1 -> Enabled Subsystem/Enable  "<enable>"
  Bus Selector/2 -> Enabled Subsystem/1(In1)  "<direction>"
  Bus Selector1/4 -> Embedded MATLAB Function/2(direction)  "<direction>"
  Bus Selector1/1 -> Subsystem1/1(e)  "<enable>"
  Second Order Linear Actuator2/1(Ac_ac) -> Saturation/1
  t/1 -> Subsystem/1(In1)
  Bus Selector1/2 -> Subsystem1/2(u)  "<up>"
  Bus Selector1/3 -> Subsystem1/3(p)  "<period>"
  Subsystem1/1(Out1) -> Embedded MATLAB Function/1(trigger)
  [rudderAngle] -> Embedded MATLAB Function/4(resetToAngle)
  [newHilData] -> Logical Operator1/1
  [sensorOverride] -> Logical Operator1/2
  Logical Operator1/1 -> Embedded MATLAB Function/3(reset), Scope1/1
  Second Order Linear Actuator3/1(Ac_ac) -> t_d/1
  Saturation/1 -> r_d/1, To Workspace/1

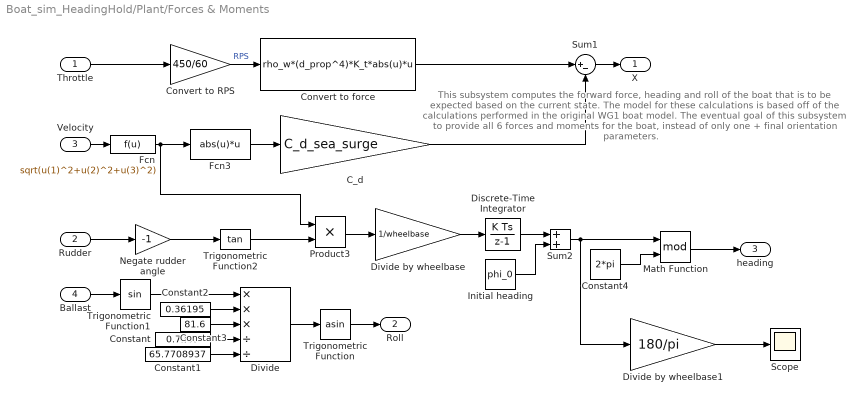
== system Boat_sim_HeadingHold/Plant/Forces & Moments ==
  note: This subsystem computes the forward force, heading and roll of the boat that
      | is to be expected based on the current state. The model for these calculations
      | is based off of the calculations performed in the original WG1 boat model.
      |
      | The eventual goal of this subsystem to provide all 6 forces and moments for the
      | boat, instead of only one + final orientation parameters.
  Throttle : Inport  OutDataType=sfix(16)  OutScaling=2^0
  Rudder : Inport  Port=2  OutDataType=sfix(16)  OutScaling=2^0
  Velocity : Inport  Port=3  OutDataType=sfix(16)  OutScaling=2^0
  Ballast : Inport  Port=4  OutDataType=sfix(16)  OutScaling=2^0
  C_d : Gain  Gain=C_d_sea_surge  ParameterDataType=sfix(16)  ParameterScaling=2^0  OutDataType=sfix(16)  OutScaling=2^0
  Constant : Constant  Value=0.7239  OutDataType=sfix(16)  OutScaling=2^0
  Constant1 : Constant  Value=65.7708937  OutDataType=sfix(16)  OutScaling=2^0
  Constant2 : Constant  Value=0.36195  OutDataType=sfix(16)  OutScaling=2^0
  Constant3 : Constant  Value=81.6  OutDataType=sfix(16)  OutScaling=2^0
  Constant4 : Constant  Value=2*pi  OutDataType=fixdt(1, 16)  OutScaling=2^0
  Convert to RPS : Gain  Gain=450/60  ParameterDataType=sfix(16)  ParameterScaling=2^0  OutDataType=sfix(16)  OutScaling=2^0
  Convert to force : Fcn  Expr=rho_w*(d_prop^4)*K_t*abs(u)*u
  Discrete-Time Integrator : DiscreteIntegrator  SampleTime=.01  OutDataType=fixdt(1, 16)  OutScaling=2^0  ICPrevOutput=DiscIntNeverNeededParam  ICPrevScaledInput=DiscIntNeverNeededParam
  Divide : Product  Inputs=***//  OutDataType=sfix(16)  OutScaling=2^-10
  Divide by wheelbase : Gain  Gain=1/wheelbase  ParameterDataType=sfix(16)  ParameterScaling=2^0  OutDataType=sfix(16)  OutScaling=2^0
  Divide by wheelbase1 : Gain  Gain=180/pi  ParameterDataType=sfix(16)  ParameterScaling=2^0  OutDataType=sfix(16)  OutScaling=2^0
  Fcn : Fcn  Expr=sqrt(u(1)^2+u(2)^2+u(3)^2)
  Fcn3 : Fcn  Expr=abs(u)*u
  Initial heading : Constant  Value=phi_0  OutDataType=sfix(16)  OutScaling=2^0
  Math Function : Math  Operator=mod  OutDataType=fixdt(1, 16)  OutScaling=2^0  SaturateOnIntegerOverflow=on
  Negate rudder angle : Gain  Gain=-1  ParameterDataType=sfix(16)  ParameterScaling=2^0  OutDataType=sfix(16)  OutScaling=2^0
  Product3 : Product  OutDataType=sfix(16)  OutScaling=2^0  RndMeth=Zero
  Scope : Scope
      settings: YMin=-0.01  YMax=0.055  SaveName=ScopeData3
  Sum1 : Sum  Inputs=|+-  OutDataType=sfix(16)  OutScaling=2^0
  Sum2 : Sum  OutDataTypeMode=double  OutDataType=sfix(16)  OutScaling=2^0  OutDataTypeStr=double
  Trigonometric Function : Trigonometry  Operator=asin
  Trigonometric Function1 : Trigonometry
  Trigonometric Function2 : Trigonometry  Operator=tan  OutputSignalType=real
  X : Outport  OutDataType=sfix(16)  OutScaling=2^0
  Roll : Outport  Port=2  OutDataType=sfix(16)  OutScaling=2^0
  heading : Outport  Port=3  OutDataType=sfix(16)  OutScaling=2^0
  wires:
  Convert to RPS/1 -> Convert to force/1  "RPS"
  Fcn3/1 -> C_d/1
  Convert to force/1 -> Sum1/1
  Velocity/1 -> Fcn/1
  Throttle/1 -> Convert to RPS/1
  Sum1/1 -> X/1
  Rudder/1 -> Negate rudder angle/1
  Ballast/1 -> Trigonometric Function1/1
  Trigonometric Function1/1 -> Divide/1
  Constant2/1 -> Divide/2
  Constant3/1 -> Divide/3
  Constant/1 -> Divide/4
  Constant1/1 -> Divide/5
  Divide/1 -> Trigonometric Function/1
  Trigonometric Function/1 -> Roll/1
  Trigonometric Function2/1 -> Product3/2
  Product3/1 -> Divide by wheelbase/1
  Divide by wheelbase/1 -> Discrete-Time Integrator/1
  Discrete-Time Integrator/1 -> Sum2/1
  Fcn/1 -> Product3/1, Fcn3/1
  C_d/1 -> Sum1/2
  Negate rudder angle/1 -> Trigonometric Function2/1
  Math Function/1 -> heading/1
  Constant4/1 -> Math Function/2
  Divide by wheelbase1/1 -> Scope/1
  Sum2/1 -> Math Function/1, Divide by wheelbase1/1
  Initial heading/1 -> Sum2/2

== system Boat_sim_HeadingHold/Plant/Generate sensor data from actuator position ==
  note: Rudder sensor data is generated here. Given the ADC configuration onboard the dsPIC
      | as well as the range of voltage values for the rudder pot. the output range should be
      | <=313 for starboard, >=620 for port, and 475<=center<=505. It's mapped from the -+.7854
      | (45deg) range that is used in calculations. The rudder follow the standard right-hand-rule
      | convention and as such +1 corresponds to port and -1 corresponds to starboard.
  note: Limits are set to within 2.5% of the real physical limits. This should
      | provide enough buffer for the real system to handle it. These might want to be changed
      | to actually be closer to the real limit. The potentiometer data gives the controller a good
      | sense of where the actuators are so the limits are just emergency triggers.
  throttle : Inport  OutDataType=fixdt(1, 16)  OutScaling=2^0
  ballast : Inport  Port=2  OutDataType=fixdt(1, 16)  OutScaling=2^0
  rudder : Inport  Port=3  OutDataType=fixdt(1, 16)  OutScaling=2^0
  Bus Creator : BusCreator  Inputs=3
  Bus Creator1 : BusCreator  Inputs=3
  Compare To Constant : simulink/Logic and Bit Operations/Compare To Constant  SystemSampleTime=-1  relop=>=  const=.975  LogicOutDataTypeMode=boolean
  Compare To Constant1 : simulink/Logic and Bit Operations/Compare To Constant  SystemSampleTime=-1  relop=<=  const=-.975  LogicOutDataTypeMode=boolean
  Compare To Constant2 : simulink/Logic and Bit Operations/Compare To Constant  SystemSampleTime=-1  relop=<  const=363  LogicOutDataTypeMode=boolean
  Compare To Constant3 : simulink/Logic and Bit Operations/Compare To Constant  SystemSampleTime=-1  relop=>  const=638  LogicOutDataTypeMode=boolean
  Map from +-.7854 to [347:655] : Subsystem
  Map from -1..1 to -1023..1023 : Subsystem
  Map from -1..1 to 620..313 : Subsystem
  Throttle sensors : Outport  OutDataType=fixdt(1, 16)  OutScaling=2^0
  Ballast sensors : Outport  Port=2  OutDataType=fixdt(1, 16)  OutScaling=2^0
  Rudder sensors : Outport  Port=3  OutDataType=fixdt(1, 16)  OutScaling=2^0
  wires:
  throttle/1 -> Map from -1..1 to -1023..1023/1(In1)
  Bus Creator/1 -> Ballast sensors/1
  Compare To Constant1/1 -> Bus Creator/3  "limit starboard"
  Compare To Constant/1 -> Bus Creator/2  "limit port"
  ballast/1 -> Map from -1..1 to 620..313/1(In1), Compare To Constant/1, Compare To Constant1/1
  Bus Creator1/1 -> Rudder sensors/1
  Compare To Constant3/1 -> Bus Creator1/3  "limit starboard"
  Compare To Constant2/1 -> Bus Creator1/2  "limit port"
  rudder/1 -> Map from +-.7854 to [347:655]/1(In1)
  Map from +-.7854 to [347:655]/1(Out1) -> Bus Creator1/1, Compare To Constant2/1, Compare To Constant3/1  "position"
  Map from -1..1 to 620..313/1(Out1) -> Bus Creator/1  "position"
  Map from -1..1 to -1023..1023/1(Out1) -> Throttle sensors/1

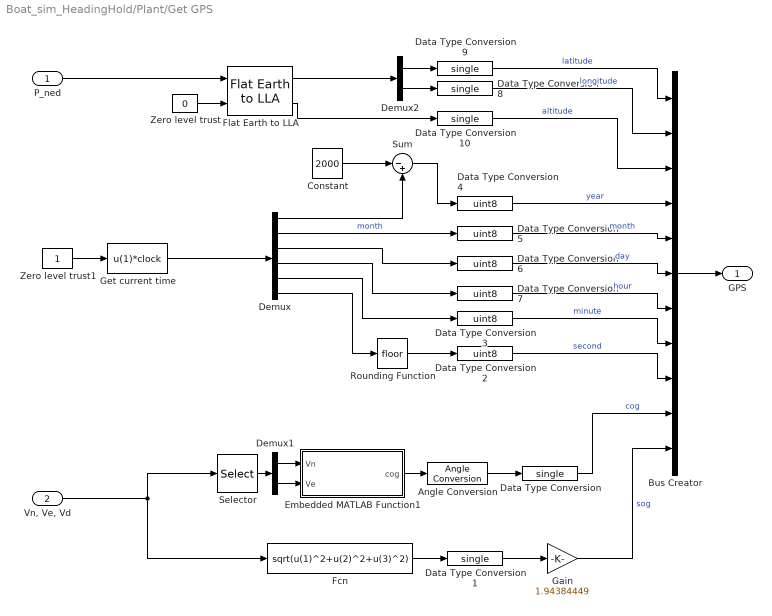
== system Boat_sim_HeadingHold/Plant/Get GPS ==
  P_ned : Inport  OutDataType=sfix(16)  OutScaling=2^0
  "Vn, Ve, Vd" : Inport  Port=2  OutDataType=sfix(16)  OutScaling=2^0
  Angle Conversion : uSimLib/Conversions/Angle Conversion  SystemSampleTime=-1  iu=rad  ou=deg
  Bus Creator : BusCreator  Inputs=11  NonVirtualBus=on
      settings: BusObject=GPS
  Constant : Constant  Value=2000  OutDataTypeMode=uint16  OutDataType=sfix(16)  OutScaling=2^0  OutDataTypeStr=uint16
  Data Type Conversion{,1,8..10} (5 alike) : DataTypeConversion  OutDataTypeMode=single  OutDataType=fixdt(1, 16)  OutScaling=2^0  OutDataTypeStr=single
  Data Type Conversion{2..7} (6 alike) : DataTypeConversion  OutDataTypeMode=uint8  OutDataType=fixdt(1, 16)  OutScaling=2^0  OutDataTypeStr=uint8
  Demux : Demux  Outputs=6
  Demux1 : Demux  Outputs=2
  Demux2 : Demux  Outputs=2
  Embedded MATLAB Function1 : Stateflow chart  TreatAsAtomicUnit=on
  Fcn : Fcn  Expr=sqrt(u(1)^2+u(2)^2+u(3)^2)
  Flat Earth to LLA : aerolibtransform2/Flat Earth to LLA  SystemSampleTime=-1  units=Metric (MKS)  ptype=Earth (WGS84)  F=1/298.257223563  R=6378137  LL0=initial_LL  psi=0
  Gain : Gain  Gain=1.94384449  ParameterDataType=fixdt(1, 16)  ParameterScaling=2^0  OutDataType=fixdt(1, 16)  OutScaling=2^0
  Get current time : MATLABFcn  MATLABFcn=u(1)*clock  OutputSignalType=real  SampleTime=T_step
  Rounding Function : Rounding
  Selector : Selector  InputPortWidth=3  IndexOptions=Index vector (dialog)  Indices=[2 1]  OutputSizes=1
  Sum : Sum  Inputs=|-+  OutDataType=sfix(16)  OutScaling=2^0
  Zero level trust : Constant  Value=0  OutDataType=sfix(16)  OutScaling=2^0
  Zero level trust1 : Constant  OutDataType=sfix(16)  OutScaling=2^0
  GPS : Outport  OutDataType=fixdt(1, 16)  OutScaling=2^0
  wires:
  Zero level trust/1 -> Flat Earth to LLA/2
  P_ned/1 -> Flat Earth to LLA/1
  Flat Earth to LLA/1 -> Demux2/1
  Flat Earth to LLA/2 -> Data Type Conversion10/1
  Demux/2 -> Data Type Conversion5/1  "month"
  Demux/3 -> Data Type Conversion6/1
  Demux/4 -> Data Type Conversion7/1
  Demux/5 -> Data Type Conversion3/1
  Demux/6 -> Rounding Function/1
  Rounding Function/1 -> Data Type Conversion2/1
  Demux2/1 -> Data Type Conversion9/1
  Demux2/2 -> Data Type Conversion8/1
  Fcn/1 -> Data Type Conversion1/1
  "Vn, Ve, Vd"/1 -> Fcn/1, Selector/1
  Embedded MATLAB Function1/1(cog) -> Angle Conversion/1
  Angle Conversion/1 -> Data Type Conversion/1
  Demux/1 -> Sum/2
  Constant/1 -> Sum/1
  Sum/1 -> Data Type Conversion4/1
  Zero level trust1/1 -> Get current time/1
  Bus Creator/1 -> GPS/1
  Data Type Conversion/1 -> Bus Creator/10  "cog"
  Data Type Conversion1/1 -> Gain/1
  Data Type Conversion2/1 -> Bus Creator/9  "second"
  Data Type Conversion3/1 -> Bus Creator/8  "minute"
  Data Type Conversion4/1 -> Bus Creator/4  "year"
  Data Type Conversion5/1 -> Bus Creator/5  "month"
  Data Type Conversion6/1 -> Bus Creator/6  "day"
  Data Type Conversion7/1 -> Bus Creator/7  "hour"
  Get current time/1 -> Demux/1
  Gain/1 -> Bus Creator/11  "sog"
  Data Type Conversion8/1 -> Bus Creator/2  "longitude"
  Data Type Conversion9/1 -> Bus Creator/1  "latitude"
  Data Type Conversion10/1 -> Bus Creator/3  "altitude"
  Selector/1 -> Demux1/1
  Demux1/1 -> Embedded MATLAB Function1/1(Vn)
  Demux1/2 -> Embedded MATLAB Function1/2(Ve)

== system Boat_sim_HeadingHold/Plant/Outputs ==
  note: This subsystem converts the heading and forward forces into a position and velocity,
      | both of which are in a North-East-Down coordinate frame.
  X : Inport  OutDataType=sfix(16)  OutScaling=2^0
  heading : Inport  Port=2  OutDataType=sfix(16)  OutScaling=2^0
  Constant : Constant  Value=0  OutDataType=fixdt(1, 16)  OutScaling=2^0
  Convert to acceleration : Gain  Gain=1/mass  ParameterDataType=sfix(16)  ParameterScaling=2^0  OutDataType=sfix(16)  OutScaling=2^0
  Discrete-Time Integrator1 : DiscreteIntegrator  SampleTime=-1  OutDataType=fixdt(1, 16)  OutScaling=2^0  UpperSaturationLimit=1  LowerSaturationLimit=-1  ICPrevOutput=DiscIntNeverNeededParam  ICPrevScaledInput=DiscIntNeverNeededParam
  Discrete-Time Integrator2 : DiscreteIntegrator  SampleTime=-1  OutDataType=fixdt(1, 16)  OutScaling=2^0  UpperSaturationLimit=1  LowerSaturationLimit=-1  ICPrevOutput=DiscIntNeverNeededParam  ICPrevScaledInput=DiscIntNeverNeededParam
  Matrix Concatenate : Concatenate  NumInputs=3  Mode=Vector
  Product1 : Product  OutDataType=sfix(16)  OutScaling=2^0  RndMeth=Zero
  Product3 : Product  OutDataType=sfix(16)  OutScaling=2^0  RndMeth=Zero
  Trigonometric Function1 : Trigonometry  OutputSignalType=real
  Trigonometric Function2 : Trigonometry  Operator=cos  OutputSignalType=real
  position : Outport  OutDataType=sfix(16)  OutScaling=2^0
  Velocity : Outport  Port=2  OutDataType=sfix(16)  OutScaling=2^0
  wires:
  Convert to acceleration/1 -> Discrete-Time Integrator2/1
  Discrete-Time Integrator2/1 -> Product3/1, Product1/1
  heading/1 -> Trigonometric Function2/1, Trigonometric Function1/1
  Discrete-Time Integrator1/1 -> position/1
  Trigonometric Function2/1 -> Product3/2
  Matrix Concatenate/1 -> Velocity/1, Discrete-Time Integrator1/1
  Product3/1 -> Matrix Concatenate/1
  Product1/1 -> Matrix Concatenate/2
  Trigonometric Function1/1 -> Product1/2
  Constant/1 -> Matrix Concatenate/3
  X/1 -> Convert to acceleration/1

== system Boat_sim_HeadingHold/Subsystem/Autonomous Controller ==
  note: This subsystem currently provides autonomous control of the boat. It utilizes simple PID control
      | on the throttle and rudder based on desired location and bearing. Calculations are performed
      | to compute a straight-line path between current location and the programmed waypoint. The
      | boat then sets out to achieve this course.
  GPS : Inport  OutDataType=sfix(16)  OutScaling=2^0
  sensors_t : Inport  Port=2  OutDataType=sfix(16)  OutScaling=2^0
  sensors_r : Inport  Port=3  OutDataType=sfix(16)  OutScaling=2^0
  sensors_b : Inport  Port=4  OutDataType=sfix(16)  OutScaling=2^0
  reset : Inport  Port=5  OutDataType=sfix(16)  OutScaling=2^0
  waypoints : Inport  Port=6  OutDataType=sfix(16)  OutScaling=2^0
  Ballast Command : Subsystem
  Rudder Command : Subsystem
  State Keeper & Estimator : Subsystem
  Terminator : Terminator
  Terminator1 : Terminator
  Terminator2 : Terminator
  Throttle Command : Subsystem
  Rudder command : Outport  OutDataType=sfix(16)  OutScaling=2^0
  Throttle command : Outport  Port=2  OutDataType=sfix(16)  OutScaling=2^0
  Tray angle command : Outport  Port=3  OutDataType=sfix(16)  OutScaling=2^0
  tag scope: waypoints=global
  wires:
  State Keeper & Estimator/6(heading) -> Rudder Command/4(Heading)
  waypoints/1 -> [waypoints]
  reset/1 -> Rudder Command/3(Reset), Throttle Command/2(reset), State Keeper & Estimator/3(reset)
  State Keeper & Estimator/1(sensors_t) -> Throttle Command/1(sensors)
  State Keeper & Estimator/2(sensors_r) -> Rudder Command/2(Sensors)
  State Keeper & Estimator/4(velocity) -> Rudder Command/1(Velocity)
  GPS/1 -> State Keeper & Estimator/4(gps)
  Throttle Command/1(command) -> Throttle command/1
  Rudder Command/1(Command) -> Rudder command/1
  Ballast Command/1(c_ballast) -> Tray angle command/1
  sensors_b/1 -> State Keeper & Estimator/5(ballast)
  sensors_r/1 -> State Keeper & Estimator/2(rudder)
  sensors_t/1 -> State Keeper & Estimator/1(throttle)
  State Keeper & Estimator/3(sensors_b) -> Terminator2/1
  State Keeper & Estimator/7(lla) -> Terminator/1
  State Keeper & Estimator/8(datetime) -> Terminator1/1
